simulink model "PMSM_vector_control_single_svpwm"  (R2019a)
settings: Solver=ode4  StartTime=0.0  StopTime=Tfinal  FixedStep=Ts  RelTol=1e-3  EnableMultiTasking=on
values from neighbouring files (symbols this model uses):
  Cdc = 150e-6    (= 0.00015)    [PMSM_modular_vector_control_sim_parameters.m]    (also in PMSM_vector_control_single_parameters.m)
  FaultTime = 10    [PMSM_vector_control_single_parameters.m]
  fsw = 40e3    (= 40000)    [PMSM_modular_vector_control_sim_parameters.m]    (also in PMSM_vector_control_single_parameters.m)
  IdPIDmax = Vdcm/5    (= 20)    [PMSM_modular_vector_control_sim_parameters.m]    (also in PMSM_vector_control_single_parameters.m = 54)
  IdPIDmin = -Vdcm/5    (= -20)    [PMSM_modular_vector_control_sim_parameters.m]    (also in PMSM_vector_control_single_parameters.m = -54)
  Idref = 0    [PMSM_vector_control_single_parameters.m]
  Inertia = 1e-2    (= 0.01)    [PMSM_modular_vector_control_sim_parameters.m]    (also in PMSM_vector_control_single_parameters.m)
  IqPIDmax = Vdcm-10    (= 90)    [PMSM_modular_vector_control_sim_parameters.m]    (also in PMSM_vector_control_single_parameters.m = 260)
  IqPIDmin = -(Vdcm-10)    (= -90)    [PMSM_modular_vector_control_sim_parameters.m]    (also in PMSM_vector_control_single_parameters.m = -260)
  IrefOverTref = MotorSpeedRad/(EfRated*3)    (= 0.261799387799)    [PMSM_modular_vector_control_sim_parameters.m]    (also in PMSM_vector_control_single_parameters.m)
  LoadTorque1 = 2    [PMSM_modular_vector_control_sim_parameters.m]    (also in PMSM_vector_control_single_parameters.m = 30)
  LoadTorque2 = 2    [PMSM_modular_vector_control_sim_parameters.m]    (also in PMSM_vector_control_single_parameters.m = 20)
  LoadTorqueStepTime = 3    [PMSM_modular_vector_control_sim_parameters.m]    (also in PMSM_vector_control_single_parameters.m = 0.5)
  phase = [0 0 0 0]    [PMSM_modular_vector_control_sim_parameters.m]    (also in PMSM_vector_control_single_parameters.m)
  PolePairs = 10    [PMSM_modular_vector_control_sim_parameters.m]    (also in PMSM_vector_control_single_parameters.m)
  Rin = 1e-3    (= 0.001)    [PMSM_modular_vector_control_sim_parameters.m]    (also in PMSM_vector_control_single_parameters.m)
  Rs = 321e-3    (= 0.321)    [PMSM_modular_vector_control_sim_parameters.m]    (also in PMSM_vector_control_single_parameters.m)
  SpeedPIDmax = 20    [PMSM_modular_vector_control_sim_parameters.m]    (also in PMSM_vector_control_single_parameters.m = 60)
  SpeedPIDmin = -20    [PMSM_modular_vector_control_sim_parameters.m]    (also in PMSM_vector_control_single_parameters.m = -60)
  SpeedRef1 = 200    [PMSM_modular_vector_control_sim_parameters.m]    (also in PMSM_vector_control_single_parameters.m = 600)
  SpeedRef2 = 100    [PMSM_modular_vector_control_sim_parameters.m]    (also in PMSM_vector_control_single_parameters.m = 200)
  SpeedRefStepTime = 6    [PMSM_modular_vector_control_sim_parameters.m]    (also in PMSM_vector_control_single_parameters.m = 0.5)
  Ts = 1000e-9    (= 1e-06)    [PMSM_modular_vector_control_sim_parameters.m]    (also in PMSM_vector_control_single_parameters.m)
  Vin = Vdc + Rin*(Pout/Vdc)    (= 200.01)    [PMSM_modular_vector_control_sim_parameters.m]    (also in PMSM_vector_control_single_parameters.m = 270.007407407)
  ViscousFriction = 1e-3    (= 0.001)    [PMSM_modular_vector_control_sim_parameters.m]    (also in PMSM_vector_control_single_parameters.m)
undefined symbols (not defined in the file or in its folder): Lload, Rload
libraries: powerlib x20, powerlib_meascontrol x5, simulink x4
settings Model: Creator=ugurm  LastModifiedBy=hakan
settings DataIOCC: LimitDataPoints=on  SaveFormat=Array  ReturnWorkspaceOutputs=off
settings OptimizationCC: LifeSpan=inf
settings DebuggingCC: UnderspecifiedInitializationDetection=Classic  MergeDetectMultiDrivingBlocksExec=none  SolverPrmCheckMsg=warning  StateNameClashWarn=warning  SFUnexpectedBacktrackingDiag=warning  SFNoUnconditionalDefaultTransitionDiag=warning  ArithmeticOperatorsInVariantConditions=warning
settings HardwareCC: ProdBitPerPointer=32  ProdBitPerSizeT=32  ProdBitPerPtrDiffT=32  ProdLargestAtomicFloat=None  ProdIntDivRoundTo=Undefined  ProdEndianess=Unspecified  ProdWordSize=32  ProdHWDeviceType=32-bit Generic
settings ModelReferenceCC: PropagateSignalLabelsOutOfModel=off
settings SFSimCC: SimUseLocalCustomCode=off
settings RTWCC: RTWUseLocalCustomCode=off
settings CodeAppCC: StateflowObjectComments=on
settings GRTTargetCC: TargetLangStandard=C89/C90 (ANSI)  GeneratePreprocessorConditionals=Disable all
settings ConfigComp: CovMetricSettings=dw  CovHtmlReporting=on  CovSaveCumulativeToWorkspaceVar=on  CovSaveSingleToWorkspaceVar=on  CovExternalEMLEnable=off
settings SimscapeCC: SimscapeNormalizeSystem=off

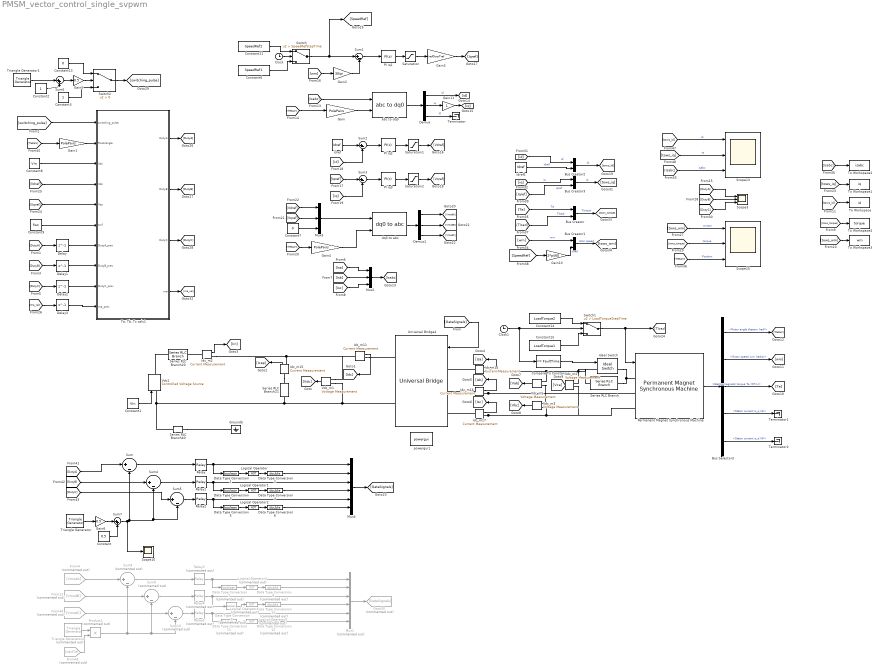
== system PMSM_vector_control_single_svpwm ==
  Bus Creator{,1..3} (4 alike) : BusCreator  Inputs=2
  Bus Selector3 : BusSelector  OutputSignals=Rotor angle thetam (rad),Rotor speed wm (rad/s),Electromagnetic torque Te (N*m),Stator current is_q (A),Stator current is_d (A)
  Clock : Clock
  Clock1 : Clock
  Compare To Constant : simulink/Logic and Bit Operations/Compare To Constant  relop=<=  const=FaultTime  OutDataTypeStr=boolean
  Constant : Constant  Value=0.5
  Constant1 : Constant  Value=Vin
  Constant11 : Constant  Value=SpeedRef2
  Constant13 : Constant  Value=0
  Constant14 : Constant  Value=LoadTorque2
  Constant15 : Constant  Value=LoadTorque1
  Constant2 : Constant
  Constant3 : Constant
  Constant6 : Constant  Value=SpeedRef1
  Constant7 : Constant  Value=0
  Constant8 : Constant  Value=Vin
  Constant9 : Constant  Value=fsw
  Data Type Conversion1 : DataTypeConversion  OutDataTypeStr=boolean
  Data Type Conversion10 : DataTypeConversion  Commented=on  OutDataTypeStr=double
  Data Type Conversion11 : DataTypeConversion  Commented=on  OutDataTypeStr=boolean
  Data Type Conversion12 : DataTypeConversion  Commented=on  OutDataTypeStr=double
  Data Type Conversion2 : DataTypeConversion  OutDataTypeStr=double
  Data Type Conversion3 : DataTypeConversion  OutDataTypeStr=boolean
  Data Type Conversion4 : DataTypeConversion  OutDataTypeStr=double
  Data Type Conversion5 : DataTypeConversion  OutDataTypeStr=boolean
  Data Type Conversion6 : DataTypeConversion  OutDataTypeStr=double
  Data Type Conversion7 : DataTypeConversion  Commented=on  OutDataTypeStr=boolean
  Data Type Conversion8 : DataTypeConversion  Commented=on  OutDataTypeStr=double
  Data Type Conversion9 : DataTypeConversion  Commented=on  OutDataTypeStr=boolean
  Delay{,1..3} (4 alike) : Delay  DelayLength=1
  Demux : Demux  Outputs=3
  Demux1 : Demux  Outputs=3
  From12 : From  Commented=on  GotoTag=VmodB
  From4 : From  Commented=on  GotoTag=VmodA
  From44 : From  Commented=on  GotoTag=VmodC
  From45 : From  Commented=on  GotoTag=VdcFilt
  Gain : Gain  Gain=PolePairs
  Gain1 : Gain  Gain=PolePairs
  Gain10 : Gain  Gain=2*pi/60
  Gain11 : Gain
  Gain2 : Gain  Gain=30/pi
  Gain3 : Gain  Gain=IrefOverTref
  Gain4 : Gain  Gain=PolePairs
  Gain5 : Gain  Gain=0.5
  Gain6 : Gain  Gain=0.5
  Goto30 : Goto  Commented=on  GotoTag=GateSignals
  Ground5 : powerlib/Elements/Ground  LConnTagsString=a
      settings: SourceProductName=Simscape Electrical
  Idc_m{2,11,14..17} (6 alike) : powerlib/Measurements/Current Measurement  PhasorSimulation=off  OutputType=Complex  PSBequivalent=0
      settings: SourceProductName=Simscape Electrical
  Ideal Switch : powerlib/Power Electronics/Ideal Switch  Ron=0.001  Lon=0  IC=0  Rs=1e5  Cs=inf  Measurements=on
      settings: SourceProductName=Simscape Electrical
  Logical Operator : Logic  Operator=NOT  AllPortsSameDT=off  OutDataTypeStr=boolean
  Logical Operator1 : Logic  Operator=NOT  AllPortsSameDT=off  OutDataTypeStr=boolean
  Logical Operator2 : Logic  Operator=NOT  AllPortsSameDT=off  OutDataTypeStr=boolean
  Logical Operator3 : Logic  Commented=on  Operator=NOT  AllPortsSameDT=off  OutDataTypeStr=boolean
  Logical Operator4 : Logic  Commented=on  Operator=NOT  AllPortsSameDT=off  OutDataTypeStr=boolean
  Logical Operator5 : Logic  Commented=on  Operator=NOT  AllPortsSameDT=off  OutDataTypeStr=boolean
  Mux1 : Mux  Commented=on  Inputs=6
  Mux2 : Mux  Inputs=3
  Mux3 : Mux  Inputs=3
  Mux4 : Mux  Inputs=6
  PI iq1 : simulink/Continuous/PID Controller  Controller=PI  Form=Parallel  TimeDomain=Discrete-time  SampleTime=-1  IntegratorMethod=Forward Euler  FilterMethod=Forward Euler  ControllerParametersSource=internal  P=0.1  I=1  D=0  UseFilter=on  N=100  TunerSelectOption=Transfer Function Based (PID Tuner App)  InitialConditionSource=internal  InitialConditionForIntegrator=0  InitialConditionForFilter=0  DifferentiatorICPrevScaledInput=0  ExternalReset=none  TrackingMode=off  Kt=1  LimitOutput=off  UpperSaturationLimit=inf  LowerSaturationLimit=-inf  LinearizeAsGain=on  AntiWindupMode=none  Kb=1  POutMin=[]  POutMax=[]  IOutMin=[]  IOutMax=[]  DOutMin=[]  DOutMax=[]  NOutMin=[]  NOutMax=[]  SumOutMin=[]  SumOutMax=[]  SaturationOutMin=[]  SaturationOutMax=[]  PParamMin=[]  PParamMax=[]  IParamMin=[]  IParamMax=[]  DParamMin=[]  DParamMax=[]  NParamMin=[]  NParamMax=[]  KbParamMin=[]  KbParamMax=[]  KtParamMin=[]  KtParamMax=[]  KbOutMin=[]  KbOutMax=[]  KtOutMin=[]  KtOutMax=[]  IntegratorOutMin=[]  IntegratorOutMax=[]  FilterOutMin=[]  FilterOutMax=[]  SumI1OutMin=[]  SumI1OutMax=[]  SumI2OutMin=[]  SumI2OutMax=[]  SumI3OutMin=[]  SumI3OutMax=[]  SumI4OutMin=[]  SumI4OutMax=[]  SumDOutMin=[]  SumDOutMax=[]  DifferentiatorOutMin=[]  DifferentiatorOutMax=[]  FilterDiffOutCoefMin=[]  FilterDiffOutCoefMax=[]  ReciprocalOutMin=[]  ReciprocalOutMax=[]  SumDenOutMin=[]  SumDenOutMax=[]  SumNumOutMin=[]  SumNumOutMax=[]  DivideOutMin=[]  DivideOutMax=[]  IntegratorContinuousStateAttributes=''  IntegratorStateMustResolveToSignalObject=off  IntegratorRTWStateStorageClass=Auto  FilterContinuousStateAttributes=''  FilterStateMustResolveToSignalObject=off  FilterRTWStateStorageClass=Auto  ParallelPVariant=InternalParameters  IdealPVariant=Disabled  IVariant=InternalParameters  DVariant=Disabled  IntegratorVariant=Discrete  SatVariant=Disabled  AWVariant=Passthrough  PCopyVariant=Disabled  TRVariant=Disabled  FdbkBlocksVariant=Forward  IdealPFdbkVariant=Disabled  SatFdbkVariant=Disabled  DerivativeFilterVariant=Disabled  NVariant=Disabled  NCopyVariant=Disabled_SignalSpec  FilterICVariant=Disabled  IntegratorICVariant=InternalICs  ExternalResetVariant=Disabled  TRSumVariant=Passthrough  SumFdbkVariant=Disabled  SumVariant=Sum_PI
  PI iq2 : simulink/Continuous/PID Controller  Controller=PI  Form=Parallel  TimeDomain=Discrete-time  SampleTime=-1  IntegratorMethod=Forward Euler  FilterMethod=Forward Euler  ControllerParametersSource=internal  P=200  I=200  D=0  UseFilter=on  N=100  TunerSelectOption=Transfer Function Based (PID Tuner App)  InitialConditionSource=internal  InitialConditionForIntegrator=0  InitialConditionForFilter=0  DifferentiatorICPrevScaledInput=0  ExternalReset=none  TrackingMode=off  Kt=1  LimitOutput=off  UpperSaturationLimit=inf  LowerSaturationLimit=-inf  LinearizeAsGain=on  AntiWindupMode=none  Kb=1  POutMin=[]  POutMax=[]  IOutMin=[]  IOutMax=[]  DOutMin=[]  DOutMax=[]  NOutMin=[]  NOutMax=[]  SumOutMin=[]  SumOutMax=[]  SaturationOutMin=[]  SaturationOutMax=[]  PParamMin=[]  PParamMax=[]  IParamMin=[]  IParamMax=[]  DParamMin=[]  DParamMax=[]  NParamMin=[]  NParamMax=[]  KbParamMin=[]  KbParamMax=[]  KtParamMin=[]  KtParamMax=[]  KbOutMin=[]  KbOutMax=[]  KtOutMin=[]  KtOutMax=[]  IntegratorOutMin=[]  IntegratorOutMax=[]  FilterOutMin=[]  FilterOutMax=[]  SumI1OutMin=[]  SumI1OutMax=[]  SumI2OutMin=[]  SumI2OutMax=[]  SumI3OutMin=[]  SumI3OutMax=[]  SumI4OutMin=[]  SumI4OutMax=[]  SumDOutMin=[]  SumDOutMax=[]  DifferentiatorOutMin=[]  DifferentiatorOutMax=[]  FilterDiffOutCoefMin=[]  FilterDiffOutCoefMax=[]  ReciprocalOutMin=[]  ReciprocalOutMax=[]  SumDenOutMin=[]  SumDenOutMax=[]  SumNumOutMin=[]  SumNumOutMax=[]  DivideOutMin=[]  DivideOutMax=[]  IntegratorContinuousStateAttributes=''  IntegratorStateMustResolveToSignalObject=off  IntegratorRTWStateStorageClass=Auto  FilterContinuousStateAttributes=''  FilterStateMustResolveToSignalObject=off  FilterRTWStateStorageClass=Auto  ParallelPVariant=InternalParameters  IdealPVariant=Disabled  IVariant=InternalParameters  DVariant=Disabled  IntegratorVariant=Discrete  SatVariant=Disabled  AWVariant=Passthrough  PCopyVariant=Disabled  TRVariant=Disabled  FdbkBlocksVariant=Forward  IdealPFdbkVariant=Disabled  SatFdbkVariant=Disabled  DerivativeFilterVariant=Disabled  NVariant=Disabled  NCopyVariant=Disabled_SignalSpec  FilterICVariant=Disabled  IntegratorICVariant=InternalICs  ExternalResetVariant=Disabled  TRSumVariant=Passthrough  SumFdbkVariant=Disabled  SumVariant=Sum_PI
  PI iq3 : simulink/Continuous/PID Controller  Controller=PI  Form=Parallel  TimeDomain=Discrete-time  SampleTime=-1  IntegratorMethod=Forward Euler  FilterMethod=Forward Euler  ControllerParametersSource=internal  P=200  I=200  D=0  UseFilter=on  N=100  TunerSelectOption=Transfer Function Based (PID Tuner App)  InitialConditionSource=internal  InitialConditionForIntegrator=0  InitialConditionForFilter=0  DifferentiatorICPrevScaledInput=0  ExternalReset=none  TrackingMode=off  Kt=1  LimitOutput=off  UpperSaturationLimit=inf  LowerSaturationLimit=-inf  LinearizeAsGain=on  AntiWindupMode=none  Kb=1  POutMin=[]  POutMax=[]  IOutMin=[]  IOutMax=[]  DOutMin=[]  DOutMax=[]  NOutMin=[]  NOutMax=[]  SumOutMin=[]  SumOutMax=[]  SaturationOutMin=[]  SaturationOutMax=[]  PParamMin=[]  PParamMax=[]  IParamMin=[]  IParamMax=[]  DParamMin=[]  DParamMax=[]  NParamMin=[]  NParamMax=[]  KbParamMin=[]  KbParamMax=[]  KtParamMin=[]  KtParamMax=[]  KbOutMin=[]  KbOutMax=[]  KtOutMin=[]  KtOutMax=[]  IntegratorOutMin=[]  IntegratorOutMax=[]  FilterOutMin=[]  FilterOutMax=[]  SumI1OutMin=[]  SumI1OutMax=[]  SumI2OutMin=[]  SumI2OutMax=[]  SumI3OutMin=[]  SumI3OutMax=[]  SumI4OutMin=[]  SumI4OutMax=[]  SumDOutMin=[]  SumDOutMax=[]  DifferentiatorOutMin=[]  DifferentiatorOutMax=[]  FilterDiffOutCoefMin=[]  FilterDiffOutCoefMax=[]  ReciprocalOutMin=[]  ReciprocalOutMax=[]  SumDenOutMin=[]  SumDenOutMax=[]  SumNumOutMin=[]  SumNumOutMax=[]  DivideOutMin=[]  DivideOutMax=[]  IntegratorContinuousStateAttributes=''  IntegratorStateMustResolveToSignalObject=off  IntegratorRTWStateStorageClass=Auto  FilterContinuousStateAttributes=''  FilterStateMustResolveToSignalObject=off  FilterRTWStateStorageClass=Auto  ParallelPVariant=InternalParameters  IdealPVariant=Disabled  IVariant=InternalParameters  DVariant=Disabled  IntegratorVariant=Discrete  SatVariant=Disabled  AWVariant=Passthrough  PCopyVariant=Disabled  TRVariant=Disabled  FdbkBlocksVariant=Forward  IdealPFdbkVariant=Disabled  SatFdbkVariant=Disabled  DerivativeFilterVariant=Disabled  NVariant=Disabled  NCopyVariant=Disabled_SignalSpec  FilterICVariant=Disabled  IntegratorICVariant=InternalICs  ExternalResetVariant=Disabled  TRSumVariant=Passthrough  SumFdbkVariant=Disabled  SumVariant=Sum_PI
  Permanent Magnet Synchronous Machine : powerlib/Machines/Permanent Magnet Synchronous Machine  NbPhases=3  FluxDistribution=Sinusoidal  RotorType=Round  MechanicalLoad=Torque Tm  PresetModel=No  ShowDetailedParameters=on  MeasurementBus=off  Resistance=Rs  Inductance=8.5e-3  dqInductances=[3.1e-3,3.6e-3]  La=Ls  MachineConstant=Voltage Constant (V_peak L-L / krpm)  Flux=0.18006  VoltageCst=VoltageConstant  TorqueCst=2.7009  Flat=120  Mechanical=[Inertia ViscousFriction PolePairs 0]  PolePairs=4  InitialConditions=[0,0, 0,0]  InitialConditions5ph=[0 0 0 0 0 0]  TsPowergui=0  TsBlock=-1  RefAngle=90 degrees behind phase A axis (modified Park)
  Product1 : Product  Commented=on
  Relay : Relay
  Relay1 : Relay
  Relay2 : Relay
  Relay3 : Relay  Commented=on
  Relay4 : Relay  Commented=on
  Relay5 : Relay  Commented=on
  Saturation : Saturate  UpperLimit=SpeedPIDmax  LowerLimit=SpeedPIDmin
  Saturation1 : Saturate  UpperLimit=IdPIDmax  LowerLimit=IdPIDmin
  Saturation2 : Saturate  UpperLimit=IqPIDmax  LowerLimit=IqPIDmin
  Scope10 : Scope
  Scope13 : Scope  NumInputPorts=3
  Scope15 : Scope  NumInputPorts=3
  Scope3 : Scope  NumInputPorts=3
  Series RLC Branch : powerlib/Elements/Series RLC Branch  LConnTagsString=__new0  RConnTagsString=__new0  BranchType=R  Resistance=5000  Inductance=1e-3  SetiL0=off  InitialCurrent=0  Capacitance=1e-6  Setx0=off  InitialVoltage=0  Measurements=None
      settings: SourceProductName=Simscape Electrical
  Series RLC Branch20 : powerlib/Elements/Series RLC Branch  LConnTagsString=__new0  RConnTagsString=__new0  BranchType=R  Resistance=Rin  Inductance=1e-3  SetiL0=off  InitialCurrent=0  Capacitance=1e-6  Setx0=off  InitialVoltage=0  Measurements=None
      settings: SourceProductName=Simscape Electrical
  Series RLC Branch21 : powerlib/Elements/Series RLC Branch  LConnTagsString=__new0  RConnTagsString=__new0  BranchType=C  Resistance=Rload  Inductance=Lload  SetiL0=off  InitialCurrent=0  Capacitance=Cdc  Setx0=off  InitialVoltage=0  Measurements=None
      settings: SourceProductName=Simscape Electrical
  Series RLC Branch40 : powerlib/Elements/Series RLC Branch  LConnTagsString=__new0  RConnTagsString=__new0  BranchType=R  Resistance=1e12  Inductance=Lload  SetiL0=off  InitialCurrent=0  Capacitance=1e-6  Setx0=off  InitialVoltage=0  Measurements=None
      settings: SourceProductName=Simscape Electrical
  Sum{,1..5} (6 alike) : Sum  Inputs=|+-
  Sum10 : Sum  Commented=on  Inputs=|+-
  Sum6 : Sum  Inputs=|++
  Sum7 : Sum  Inputs=|++
  Sum8 : Sum  Commented=on  Inputs=|+-
  Sum9 : Sum  Commented=on  Inputs=|+-
  Switch : Switch  Criteria=u2 > Threshold  Threshold=SpeedRefStepTime
  Switch1 : Switch  Criteria=u2 > Threshold  Threshold=LoadTorqueStepTime
  Switch2 : Switch  Criteria=u2 > Threshold
  "Ta, Tb, Tc calc1" : MATLAB Function  TreatAsAtomicUnit=on
  Terminator : Terminator
  Terminator1 : Terminator
  Terminator2 : Terminator
  To Workspace : ToWorkspace  VariableName=id  SaveFormat=Timeseries  SampleTime=-1
  To Workspace1 : ToWorkspace  VariableName=iq  SaveFormat=Timeseries  SampleTime=-1
  To Workspace2 : ToWorkspace  VariableName=isabc  SaveFormat=Timeseries  SampleTime=-1
  To Workspace3 : ToWorkspace  VariableName=wm  SaveFormat=Timeseries  SampleTime=-1
  To Workspace4 : ToWorkspace  VariableName=torque  SaveFormat=Timeseries  SampleTime=-1
  Triangle Generator : powerlib_meascontrol/Pulse & Signal Generators/Triangle Generator  Freq=fsw  Phase=phase(1)  Ts=Ts
      settings: SourceProductName=Simscape Electrical
  Triangle Generator1 : powerlib_meascontrol/Pulse & Signal Generators/Triangle Generator  Freq=fsw  Phase=0  Ts=Ts
      settings: SourceProductName=Simscape Electrical
  Triangle Generator2 : powerlib_meascontrol/Pulse & Signal Generators/Triangle Generator  Commented=on  Freq=fsw  Phase=phase(1)  Ts=Ts
      settings: SourceProductName=Simscape Electrical
  Universal Bridge4 : powerlib/Power Electronics/Universal Bridge  Arms=3  SnubberResistance=1e5  SnubberCapacitance=inf  Device=IGBT / Diodes  Ron=1e-6  Lon=0  ForwardVoltages="[  0  0  ]"  ForwardVoltage=0  GTOparameters=[ 10e-6 , 20e-6 ]  IGBTparameters=[0,0]  Measurements=None  Measurements_2=None  converterType=Rectifier
      settings: SourceProductName=Simscape Electrical
  Vdc1 : powerlib/Electrical Sources/Controlled Voltage Source  Initialize=off  Source_Type=DC  Amplitude=200  Phase=0  Frequency=0  Measurements=None
      settings: SourceProductName=Simscape Electrical
  Vdc_m{1..3,5} (4 alike) : powerlib/Measurements/Voltage Measurement  PhasorSimulation=off  OutputType=Complex  PSBequivalent=0
      settings: SourceProductName=Simscape Electrical
  abc to dq0 : powerlib_meascontrol/Transformations/abc to dq0  Alignment=90 degrees behind phase A axis
      settings: SourceProductName=Simscape Electrical
  dq0 to abc : powerlib_meascontrol/Transformations/dq0 to abc  Alignment=90 degrees behind phase A axis
      settings: SourceProductName=Simscape Electrical
  idref : Constant  Value=Idref
  idref1 : Constant  Value=Idref
  powergui1 : powerlib/powergui  Priority=1  SimulationMode=Discrete  SampleTime=Ts  frequency=60  Iterations=50  frequencyindice=0  Pbase=100e6  ErrMax=1e-4  UnitsV=kV  UnitsW=MW  buscounter=0  FunctionMessages=off  echomessages=off  EnableUseOfTLC=off  CurrentSourceSwitches=off  DisableSnubberDevices=off  DisableRonSwitches=off  DisableVfSwitches=off  DisplayEquations=off  AutomaticDiscreteSolvers=off  SolverType=Tustin  Interpol=off  ExternalGateDelay=off  methode=off  Ts=0  x0status=blocks  SPID=off  SwTol=0  HookPort=off  NonlinearTolerance=0  nMaxIteration=15  ContinueOnMaxIteration=off  RestoreLinks=warning  ResistiveCurrentMeasurement=off  Frange=[0:2:500]  Ylog=off  Xlog=on  ShowGrid=off  save=off  variable=ZData  structure=Icap  ZoomFFT=off  StartTime=0.04  cycles=5  DisplayStyle=3  fundamental=150  FreqAxis=off  MaxFrequency=1000  frequencyindicesteady=1  RmsSteady=1  display=off
      settings: SourceProductName=Simscape Electrical
  wires:
  Idc_m14/1 -> [Isa]
  Constant1/1 -> Vdc1/1
  Idc_m15/1 -> [Icap]
  Idc_m16/1 -> [Isb]
  Idc_m17/1 -> [Isc]
  Idc_m11/1 -> [Idc]
  Vdc_m1/1 -> [Vdc]
  Idc_m2/1 -> [Iin]
  Vdc_m5/1 -> [Vab]
  Vdc_m3/1 -> [Vbc]
  Vdc_m2/1 -> [Vca]
  [Isa] -> Mux2/1
  [Isb] -> Mux2/2
  [Isc] -> Mux2/3
  Permanent Magnet Synchronous Machine/1 -> Bus Selector3/1
  Bus Selector3/3 -> [Te]  "<Electromagnetic torque Te (N*m)>"
  Bus Selector3/2 -> [wm]  "<Rotor speed wm (rad/s)>"
  Bus Selector3/1 -> [Thetam]  "<Rotor angle thetam (rad)>"
  Mux2/1 -> [Isabc]
  [Isabc] -> abc to dq0/1
  Gain/1 -> abc to dq0/2
  [Thetam] -> Gain/1
  abc to dq0/1 -> Demux/1
  Demux/1 -> [id]  "id"
  Demux/2 -> Gain11/1  "iq"
  Demux/3 -> Terminator/1  "i0"
  [wm] -> Gain2/1
  Gain2/1 -> Sum1/2
  Switch/1 -> [SpeedRef], Sum1/1
  Sum1/1 -> PI iq1/1
  PI iq1/1 -> Saturation/1
  Saturation/1 -> Gain3/1
  Gain3/1 -> [Iqref]
  [id] -> Sum2/2
  Sum2/1 -> PI iq2/1
  PI iq2/1 -> Saturation1/1
  idref/1 -> Sum2/1
  [iq] -> Sum3/2
  Sum3/1 -> PI iq3/1
  PI iq3/1 -> Saturation2/1
  [Iqref] -> Sum3/1
  Saturation2/1 -> [Vqref]
  [Thetam] -> Gain4/1
  Gain4/1 -> dq0 to abc/2
  Constant7/1 -> Mux3/3
  Mux3/1 -> dq0 to abc/1
  dq0 to abc/1 -> Demux1/1
  Sum/1 -> Relay/1
  Sum4/1 -> Relay1/1
  Sum5/1 -> Relay2/1
  Data Type Conversion1/1 -> Logical Operator/1
  Logical Operator/1 -> Data Type Conversion2/1
  Data Type Conversion2/1 -> Mux4/2
  Data Type Conversion3/1 -> Logical Operator1/1
  Relay1/1 -> Data Type Conversion3/1, Mux4/3
  Logical Operator1/1 -> Data Type Conversion4/1
  Data Type Conversion4/1 -> Mux4/4
  Data Type Conversion5/1 -> Logical Operator2/1
  Relay2/1 -> Data Type Conversion5/1, Mux4/5
  Logical Operator2/1 -> Data Type Conversion6/1
  Data Type Conversion6/1 -> Mux4/6
  Relay/1 -> Mux4/1, Data Type Conversion1/1
  [DutyC] -> Sum5/1
  Demux1/1 -> [VmodA]
  Demux1/2 -> [VmodB]
  Demux1/3 -> [VmodC]
  Mux4/1 -> [GateSignals]
  Switch1/1 -> [Tload], Permanent Magnet Synchronous Machine/1
  [GateSignals] -> Universal Bridge4/1
  Triangle Generator/1 -> Gain6/1
  Gain11/1 -> [iq]
  Bus Selector3/4 -> Terminator1/1  "<Stator current is_q (A)>"
  Bus Selector3/5 -> Terminator2/1  "<Stator current is_d (A)>"
  Saturation1/1 -> [Vdref]
  [Vqref] -> Mux3/2
  [Vdref] -> Mux3/1
  Clock/1 -> Switch/2
  Constant11/1 -> Switch/1
  Constant6/1 -> Switch/3
  Clock1/1 -> Compare To Constant/1, Switch1/2
  Constant14/1 -> Switch1/1
  Constant15/1 -> Switch1/3
  [DutyA] -> Sum/1
  [DutyB] -> Sum4/1
  Bus Creator3/1 -> [tows_iq]  "iq"
  [Isabc] -> Scope13/3  "isabc"
  [Thetam] -> Scope15/3  "Position"
  Compare To Constant/1 -> Ideal Switch/1
  [Te] -> Bus Creator/1  "Te"
  [Tload] -> Bus Creator/2  "Tload"
  Bus Creator/1 -> [tows_torque]  "Torque"
  Bus Creator1/1 -> [tows_wm]  "rotor speed"
  [wm] -> Bus Creator1/1  "wm"
  [SpeedRef] -> Gain10/1
  idref1/1 -> Bus Creator2/2  "idref"
  [id] -> Bus Creator2/1  "id"
  Bus Creator2/1 -> [tows_id]  "id"
  [iq] -> Bus Creator3/1  "iq"
  [Iqref] -> Bus Creator3/2  "iqref"
  Gain10/1 -> Bus Creator1/2  "wref"
  "Ta, Tb, Tc calc1"/4(ma) -> [ma_val]
  Constant9/1 -> "Ta, Tb, Tc calc1"/6(swf)
  Delay/1 -> "Ta, Tb, Tc calc1"/7(DutyA_prev)
  Gain5/1 -> Switch2/2
  Constant2/1 -> Sum6/2
  "Ta, Tb, Tc calc1"/1(DutyA) -> [DutyA]
  Constant3/1 -> Switch2/3
  Constant13/1 -> Switch2/1
  [DutyC] -> Delay2/1
  Triangle Generator1/1 -> Sum6/1
  Switch2/1 -> [switching_pulse]
  Constant8/1 -> "Ta, Tb, Tc calc1"/3(Vdc)
  [switching_pulse] -> "Ta, Tb, Tc calc1"/1(switching_pulse)
  Delay1/1 -> "Ta, Tb, Tc calc1"/8(DutyB_prev)
  Delay2/1 -> "Ta, Tb, Tc calc1"/9(DutyC_prev)
  "Ta, Tb, Tc calc1"/3(DutyC) -> [DutyC]
  "Ta, Tb, Tc calc1"/2(DutyB) -> [DutyB]
  [DutyA] -> Delay/1
  Sum6/1 -> Gain5/1
  [DutyB] -> Delay1/1
  [Thetam] -> Gain1/1
  [DutyC] -> Scope3/3
  [DutyA] -> Scope3/1
  [DutyB] -> Scope3/2
  Gain6/1 -> Sum7/1
  Sum7/1 -> Scope10/1, Sum5/2, Sum4/2, Sum/2
  Constant/1 -> Sum7/2
  Sum10/1 -> Relay5/1
  Logical Operator4/1 -> Data Type Conversion10/1
  From45/1 -> Product1/2
  Sum9/1 -> Relay4/1
  Relay5/1 -> Data Type Conversion11/1, Mux1/5
  Data Type Conversion12/1 -> Mux1/6
  Product1/1 -> Sum8/2, Sum9/2, Sum10/2
  Data Type Conversion7/1 -> Logical Operator3/1
  From44/1 -> Sum10/1
  Mux1/1 -> Goto30/1
  Logical Operator3/1 -> Data Type Conversion8/1
  Sum8/1 -> Relay3/1
  Relay4/1 -> Data Type Conversion9/1, Mux1/3
  Data Type Conversion8/1 -> Mux1/2
  From4/1 -> Sum8/1
  Data Type Conversion9/1 -> Logical Operator4/1
  Logical Operator5/1 -> Data Type Conversion12/1
  Data Type Conversion10/1 -> Mux1/4
  Relay3/1 -> Mux1/1, Data Type Conversion7/1
  Data Type Conversion11/1 -> Logical Operator5/1
  Triangle Generator2/1 -> Product1/1
  From12/1 -> Sum9/1
  [ma_val] -> Delay3/1
  Delay3/1 -> "Ta, Tb, Tc calc1"/10(ma_prev)
  [tows_torque] -> To Workspace4/1
  [tows_wm] -> To Workspace3/1
  [tows_id] -> To Workspace/1
  [tows_iq] -> To Workspace1/1
  [tows_wm] -> Scope15/1  "wrotor"
  [tows_torque] -> Scope15/2  "torque"
  [Isabc] -> To Workspace2/1
  [tows_id] -> Scope13/1  "id"
  [tows_iq] -> Scope13/2  "iq"
  Gain1/1 -> "Ta, Tb, Tc calc1"/2(RotorAngle)
  [Vdref] -> "Ta, Tb, Tc calc1"/4(Vds)
  [Vqref] -> "Ta, Tb, Tc calc1"/5(Vqs)
  connections:
  Vdc_m5/LConn1 -- Series RLC Branch/LConn1 -- Ideal Switch/LConn1 -- Vdc_m2/LConn2 -- Idc_m14/RConn1
  Series RLC Branch40/RConn1 -- Ground5/LConn1
  Idc_m14/LConn1 -- Universal Bridge4/LConn1
  Idc_m15/LConn1 -- Series RLC Branch21/LConn1
  Vdc1/RConn1 -- Series RLC Branch20/LConn1
  Idc_m16/LConn1 -- Universal Bridge4/LConn2
  Idc_m17/LConn1 -- Universal Bridge4/LConn3
  Idc_m17/RConn1 -- Permanent Magnet Synchronous Machine/LConn3 -- Vdc_m2/LConn1 -- Vdc_m3/LConn2
  Idc_m16/RConn1 -- Permanent Magnet Synchronous Machine/LConn2 -- Vdc_m3/LConn1 -- Vdc_m5/LConn2
  Idc_m15/RConn1 -- Idc_m11/LConn1 -- Vdc_m1/LConn1 -- Idc_m2/RConn1
  Idc_m11/RConn1 -- Universal Bridge4/RConn1
  Vdc_m1/LConn2 -- Universal Bridge4/RConn2 -- Series RLC Branch21/RConn1 -- Vdc1/LConn1 -- Series RLC Branch40/LConn1
  Idc_m2/LConn1 -- Series RLC Branch20/RConn1
  Ideal Switch/RConn1 -- Series RLC Branch/RConn1 -- Permanent Magnet Synchronous Machine/LConn1

== matlab function PMSM_vector_control_single_svpwm/Ta, Tb, Tc calc1 ==
  data: switching_pulse input; RotorAngle input; Vdc input; Vds input; Vqs input; swf input; DutyA output; DutyB output; DutyC output; DutyA_prev input; DutyB_prev input; DutyC_prev input; ma output; ma_prev input
function [DutyA, DutyB, DutyC, ma] = fcn(switching_pulse,RotorAngle,Vdc,Vds,Vqs, swf,DutyA_prev, DutyB_prev, DutyC_prev,ma_prev)

Tsw = 1/swf;
T1 = 0;
T2 = 0;
T0 = 0;

DutyA = 0;
DutyB = 0;
DutyC = 0;
Valfa = sin(RotorAngle)*Vds+cos(RotorAngle)*Vqs;
Vbeta =-cos(RotorAngle)*Vds+sin(RotorAngle)*Vqs;
VoltageVectorAngle = atan2(Vbeta,Valfa)+4*pi;

sectornumber = 0;
VoltageVectorAngleAlfa = mod(VoltageVectorAngle,pi/3);


if(switching_pulse==1)
    ma = sqrt(Vds^2+Vqs^2)/(Vdc/sqrt(3));
    T1 = Tsw*ma*sin(pi/3-VoltageVectorAngleAlfa);
    T2 = Tsw*ma*sin(VoltageVectorAngleAlfa);
    T0 = Tsw-T1-T2;
    if (mod(VoltageVectorAngle, 2*pi)<=pi/3)&&(mod(VoltageVectorAngle, 2*pi)>=0)  % sector 1
        DutyA = (T1+T2+T0/2)/Tsw;
        DutyB = (T2+T0/2)/Tsw;
        DutyC = (T0/2)/Tsw;
        sectornumber = 1;
        return;
    end
    if (mod(VoltageVectorAngle, 2*pi)<=2*pi/3)&&(mod(VoltageVectorAngle, 2*pi)>=pi/3)  % sector 2
        DutyA = (T1+T0/2)/Tsw;
        DutyB = (T1+T2+T0/2)/Tsw;
        DutyC = (T0/2)/Tsw;
        sectornumber = 2;
        return;
    end
    if (mod(VoltageVectorAngle, 2*pi)<=pi)&&(mod(VoltageVectorAngle, 2*pi)>=2*pi/3)  % sector 3
        if(mod(VoltageVectorAngle, pi)==0)
            DutyA = (T0/2)/Tsw;
            DutyB = (T1+T0/2)/Tsw;
            DutyC = (T1+T2+T0/2)/Tsw;
        else
            DutyA = (T0/2)/Tsw;
            DutyB = (T1+T2+T0/2)/Tsw;
            DutyC = (T2+T0/2)/Tsw;
        end
        sectornumber = 3;
        return;
    end
    if (mod(VoltageVectorAngle, 2*pi)<=4*pi/3)&&(mod(VoltageVectorAngle, 2*pi)>=pi)  % sector 4
        DutyA = (T0/2)/Tsw;
        DutyB = (T1+T0/2)/Tsw;
        DutyC = (T1+T2+T0/2)/Tsw;
        sectornumber = 4;
        return;
    end
    if (mod(VoltageVectorAngle, 2*pi)<=5*pi/3)&&(mod(VoltageVectorAngle, 2*pi)>=4*pi/3)  % sector 5
        DutyA = (T2+T0/2)/Tsw;
        DutyB = (T0/2)/Tsw;
        DutyC = (T1+T2+T0/2)/Tsw;
        sectornumber = 5;
        return;
    end
    if (mod(VoltageVectorAngle, 2*pi)<=2*pi)&&(mod(VoltageVectorAngle, 2*pi)>=5*pi/3)  % sector 6
        DutyA = (T1+T2+T0/2)/Tsw;
        DutyB = (T0/2)/Tsw;
        DutyC = (T1+T0/2)/Tsw;
        sectornumber = 6;
        return;
    end
else
    DutyA = DutyA_prev;
    DutyB = DutyB_prev;
    DutyC = DutyC_prev;
    ma = ma_prev;
end
